simulink model "model"  (R2024b)
settings: Solver=VariableStepAuto  StartTime=0.0  StopTime=10.0  RelTol=1e-3
values from neighbouring files (symbols this model uses):
  B_m = 0.3    [main.m]
  beta_e = 1e+009    (= 1000000000)    [main.m]
  D_m = 6.67E-05/(2*pi)    (= 1.06156347042e-05)    [main.m]
  J_t = 0.1    [main.m]
  p_3 = 1e5    (= 100000)    [main.m]
  q_0 = 1e-05    [main.m]
  T_L = 300    [main.m]
  V = 1.75e-3    (= 0.00175)    [main.m]
settings Model: Creator=diznutz  LastModifiedBy=diznutz

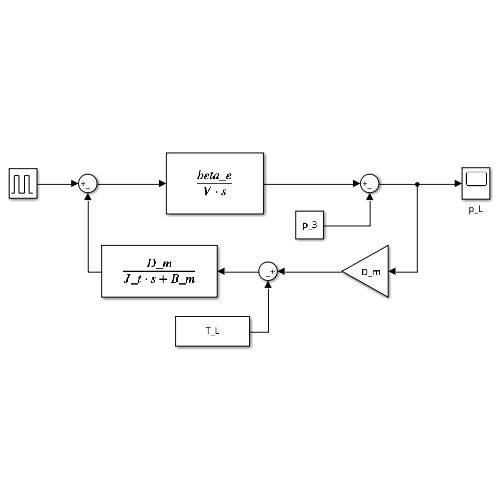
[thumbnail: Simulink's stored preview of the top-level diagram]
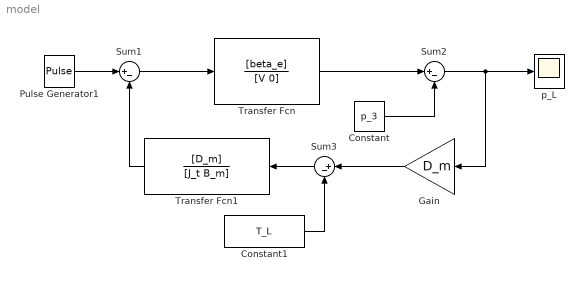
== system model ==
  Constant : Constant  Value=p_3
  Constant1 : Constant  Value=T_L
  Gain : Gain  Gain=D_m
  Pulse Generator1 : DiscretePulseGenerator  PulseType=Time based  Amplitude=q_0  Period=8  PulseWidth=25  PhaseDelay=4
  Sum1 : Sum  Inputs=|+-
  Sum2 : Sum  Inputs=|+-
  Sum3 : Sum  Inputs=|+-
  Transfer Fcn : TransferFcn  Numerator=[beta_e]  Denominator=[V 0]
  Transfer Fcn1 : TransferFcn  Numerator=[D_m]  Denominator=[J_t B_m]
  p_L : Scope
  wires:
  Sum1/1 -> Transfer Fcn/1
  Transfer Fcn/1 -> Sum2/1
  Constant/1 -> Sum2/2
  Sum2/1 -> Gain/1, p_L/1
  Constant1/1 -> Sum3/2
  Sum3/1 -> Transfer Fcn1/1
  Transfer Fcn1/1 -> Sum1/2
  Pulse Generator1/1 -> Sum1/1
  Gain/1 -> Sum3/1
